simulink model "main"  (R2021a)
settings: Solver=VariableStepAuto  StartTime=0.0  StopTime=5  RelTol=1e-3
libraries: pid_lib x1
settings Model: Creator=l.ribeiro-lustosa  LastModifiedBy=l.ribeiro-lustosa

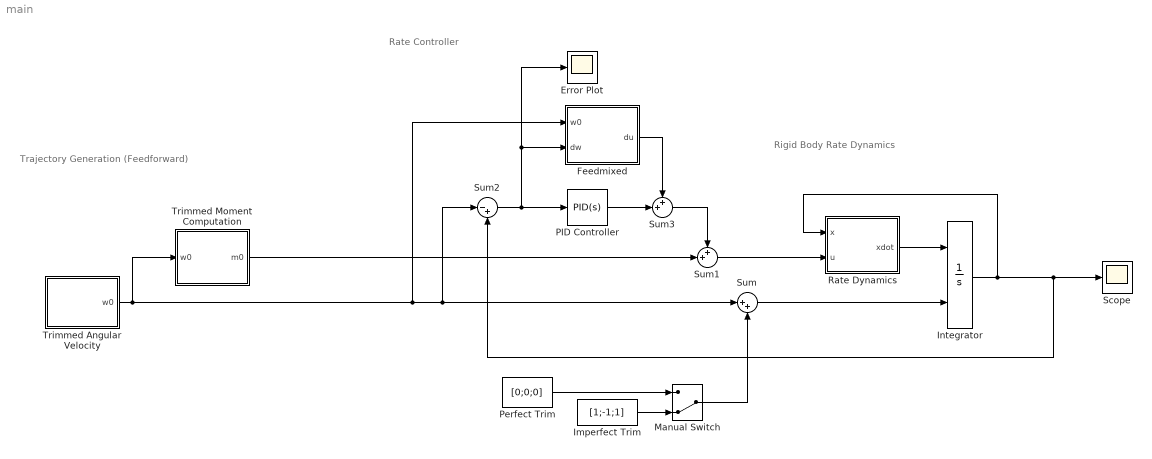
== system main ==
  note: Rate Controller
  note: Trajectory Generation (Feedforward)
  note: Rigid Body Rate Dynamics
  Error Plot : Scope
  Feedmixed : MATLAB Function  TreatAsAtomicUnit=on
  Imperfect Trim : Constant  Value=[1;-1;1]
  Integrator : Integrator  InitialConditionSource=external
  Manual Switch : ManualSwitch  CurrentSetting=0
  PID Controller : pid_lib/PID Controller  Controller=PID  Form=Parallel  TimeDomain=Continuous-time  UseExternalTs=off  SampleTime=-1  IntegratorMethod=Forward Euler  FilterMethod=Forward Euler  ControllerParametersSource=internal  P=-10  I=-1  D=0  UseFilter=on  N=100  TunerSelectOption=Frequency Response Based  InitialConditionSource=internal  InitialConditionForIntegrator=0  InitialConditionForFilter=0  DifferentiatorICPrevScaledInput=0  ExternalReset=none  TrackingMode=off  Kt=1  LimitOutput=off  SatLimitsSource=internal  UpperSaturationLimit=inf  LowerSaturationLimit=-inf  LinearizeAsGain=on  AntiWindupMode=none  Kb=1  POutMin=[]  POutMax=[]  IOutMin=[]  IOutMax=[]  DOutMin=[]  DOutMax=[]  NOutMin=[]  NOutMax=[]  SumOutMin=[]  SumOutMax=[]  SaturationOutMin=[]  SaturationOutMax=[]  PParamMin=[]  PParamMax=[]  IParamMin=[]  IParamMax=[]  DParamMin=[]  DParamMax=[]  NParamMin=[]  NParamMax=[]  KbParamMin=[]  KbParamMax=[]  KtParamMin=[]  KtParamMax=[]  KbOutMin=[]  KbOutMax=[]  KtOutMin=[]  KtOutMax=[]  IntegratorOutMin=[]  IntegratorOutMax=[]  FilterOutMin=[]  FilterOutMax=[]  SumI1OutMin=[]  SumI1OutMax=[]  SumI2OutMin=[]  SumI2OutMax=[]  SumI3OutMin=[]  SumI3OutMax=[]  SumI4OutMin=[]  SumI4OutMax=[]  SumDOutMin=[]  SumDOutMax=[]  DifferentiatorOutMin=[]  DifferentiatorOutMax=[]  FilterDiffOutCoefMin=[]  FilterDiffOutCoefMax=[]  ReciprocalOutMin=[]  ReciprocalOutMax=[]  SumDenOutMin=[]  SumDenOutMax=[]  SumNumOutMin=[]  SumNumOutMax=[]  DivideOutMin=[]  DivideOutMax=[]  UdiffTsProdOutMin=[]  UdiffTsProdOutMax=[]  NTsProdOutMin=[]  NTsProdOutMax=[]  UintegralTsProdOutMin=[]  UintegralTsProdOutMax=[]  UngainTsProdOutMin=[]  UngainTsProdOutMax=[]  IntegratorContinuousStateAttributes=''  IntegratorStateMustResolveToSignalObject=off  IntegratorRTWStateStorageClass=Auto  FilterContinuousStateAttributes=''  FilterStateMustResolveToSignalObject=off  FilterRTWStateStorageClass=Auto  ParallelPVariant=InternalParameters  IdealPVariant=Disabled  IVariant=InternalParameters  DVariant=InternalParameters  IntegratorVariant=Continuous  SatVariant=Disabled  AWVariant=Passthrough  PCopyVariant=Disabled  TRVariant=Disabled  FdbkBlocksVariant=Forward  IdealPFdbkVariant=Disabled  SatFdbkVariant=Disabled  DerivativeFilterVariant=ContFilter  NVariant=InternalParameters  NCopyVariant=Disabled  FilterICVariant=InternalICsFilter  IntegratorICVariant=InternalICs  ExternalResetVariant=Disabled  TRSumVariant=Passthrough  SumFdbkVariant=Disabled  SumVariant=Sum_PID  TsampFilterVariant=InternalTs  TsampNgainVariant=Passthrough  TsampIntegralVariant=Passthrough  ExternalSaturationOutDataTypeStr=Inherit: Same as second input
  Perfect Trim : Constant  Value=[0;0;0]
  Rate Dynamics : MATLAB Function  TreatAsAtomicUnit=on
  Scope : Scope
  Sum : Sum  Inputs=|++
  Sum1 : Sum  Inputs=++|
  Sum2 : Sum  Inputs=|-+
  Sum3 : Sum  Inputs=++|
  Trimmed Angular Velocity : MATLAB Function  TreatAsAtomicUnit=on
  Trimmed Moment Computation : MATLAB Function  TreatAsAtomicUnit=on
  wires:
  Rate Dynamics/1(xdot) -> Integrator/1
  Integrator/1 -> Sum2/2, Scope/1, Rate Dynamics/1(x)
  Trimmed Angular Velocity/1(w0) -> Sum/1, Sum2/1, Feedmixed/1(w0), Trimmed Moment Computation/1(w0)
  Sum/1 -> Integrator/2
  Perfect Trim/1 -> Manual Switch/1
  Imperfect Trim/1 -> Manual Switch/2
  Manual Switch/1 -> Sum/2
  Sum1/1 -> Rate Dynamics/2(u)
  Trimmed Moment Computation/1(m0) -> Sum1/2
  Sum2/1 -> Error Plot/1, Feedmixed/2(dw), PID Controller/1
  Sum3/1 -> Sum1/1
  PID Controller/1 -> Sum3/2
  Feedmixed/1(du) -> Sum3/1

== matlab function main/Trimmed Moment Computation ==
  data: w0 input; m0 output; J parameter
function m0 = fcn(w0,J)

m0 = cross(w0,J*w0);

== matlab function main/Rate Dynamics ==
  data: x input; u input; xdot output; J parameter
function xdot = fcn(x,u,J)

%% Newton's Second Law for Rotation
xdot = J\( u - cross(x,J*x) );

== matlab function main/Trimmed Angular Velocity ==
  data: w0 output; J parameter
function w0 = fcn(J)

%% Eigenstructure information
[V,D] = eig(J);

%% Sorting eigenvalues in ascending order
[B,I] = sort(real([D(1,1);D(2,2);D(3,3)]));

%% Choosing a principal axes as desired trimmed condition
% Notice that choosing a principal axis will yield zero actuator moment for trim
% Choice of eigenvalues:
%   i=1 --> Least eigenvalue
%   i=2 --> Intermediate Axis
%   i=3 --> Largest eigenvalue
i=2;
w0 = 10*real(V(:,I(i)));
% You can also choose a random value, but that will require nonzero
% actuator moments!!
%w0 = 10*[1;2;3];

== matlab function main/Feedmixed ==
  data: w0 input; dw input; du output; J parameter
function du = fcn(w0,dw,J)

%% model-based mixed feedback + feedforward term
du = cross( w0, J*dw );
